simulink model "discrete"  (R2017a)
settings: Solver=VariableStepAuto  StartTime=0.0  StopTime=10.0  RelTol=1e-3
undefined symbols (not defined in the file or in its folder): DCd, NCd, T
settings Model: Creator=julio  LastModifiedBy=julio
settings DataIOCC: ExternalInput=[NCd, DCd]
settings DebuggingCC: ArtificialAlgebraicLoopMsg=none

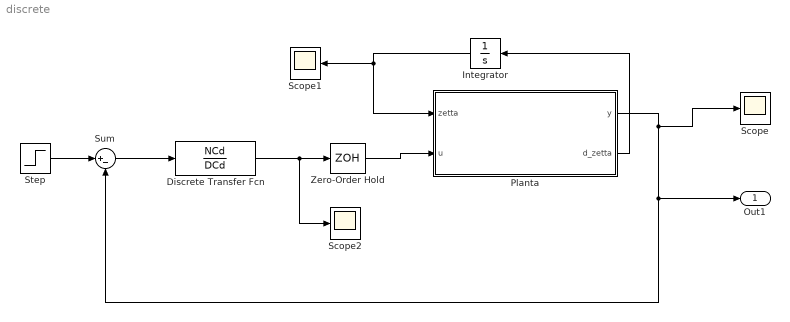
== system discrete ==
  Discrete Transfer Fcn : DiscreteTransferFcn  Numerator=NCd  Denominator=DCd  SampleTime=T  a0EqualsOne=on
  Integrator : Integrator
  Planta : MATLAB Function  TreatAsAtomicUnit=on  RTWFcnName=nonlinear_func  RTWFileName=nonlinear_func
      settings: MinAlgLoopOccurrences=on  RTWFileNameOpts=User specified
  Scope : Scope
  Scope1 : Scope
  Scope2 : Scope
  Step : Step  Time=0  After=0.3  SampleTime=0
  Sum : Sum  Inputs=|+-
  Zero-Order Hold : ZeroOrderHold  SampleTime=-1
  Out1 : Outport  SignalName=y
  wires:
  Sum/1 -> Discrete Transfer Fcn/1
  Step/1 -> Sum/1
  Zero-Order Hold/1 -> Planta/2(u)
  Planta/2(d_zetta) -> Integrator/1
  Integrator/1 -> Planta/1(zetta), Scope1/1
  Discrete Transfer Fcn/1 -> Scope2/1, Zero-Order Hold/1
  Planta/1(y) -> Scope/1, Out1/1, Sum/2

== matlab function discrete/Planta ==
  data: zetta input size=4; u input size=1; y output size=1; d_zetta output size=4
function [ y, d_zetta] = nonlinear_func(zetta, u)
%UNTITLED Summary of this function goes here
%   Detailed explanation goes here
    
    MJ = 1.0731; % [kg]
    m  = 0.209;  % [kg]
    l  = 0.3302; % [m]
    bK = 5.4;    % [N.s/(m²)]
    Kr = 1.0717; % [N/V]
    g  = 9.81;   % [m/s^2]

    M_aux = MJ + m*sin(zetta(3))^2;
    
    A = [ 0 1 0 0
          0 -bK/M_aux 0 -(m*l*zetta(4)*sin(zetta(3)))/M_aux
          0 0 0 1
          0 bK*cos(zetta(3))/(M_aux*l) 0 -m*zetta(4)*sin(zetta(3))*cos(zetta(3))/(M_aux)];
      
    F1 = m*g*sin(zetta(3))*cos(zetta(3)) + Kr*u;
    F2 = -cos(zetta(3))*F1/(l*M_aux) - g*sin(zetta(3))/l;
    
    B = [ 0 F1/M_aux 0 F2]';
    
    y = zetta(1);
    d_zetta = A*zetta + B;

end
